simulink model "Trajectories_Transpalet"  (R2022a)
settings: Solver=VariableStepAuto  StartTime=0.0  StopTime=10.0  RelTol=1e-3
libraries: roblocks x1, simulink x1
settings Model: Creator=antonio  LastModifiedBy=antonio

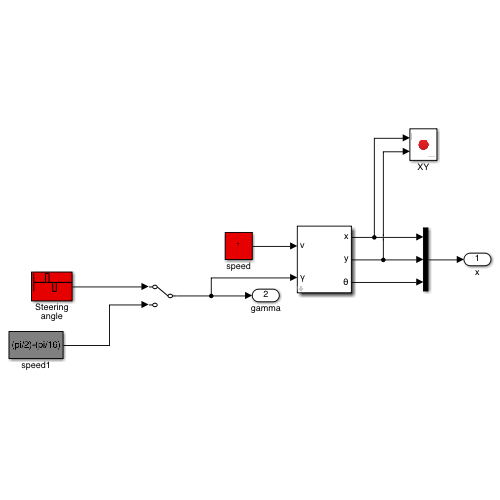
[thumbnail: Simulink's stored preview of the top-level diagram]
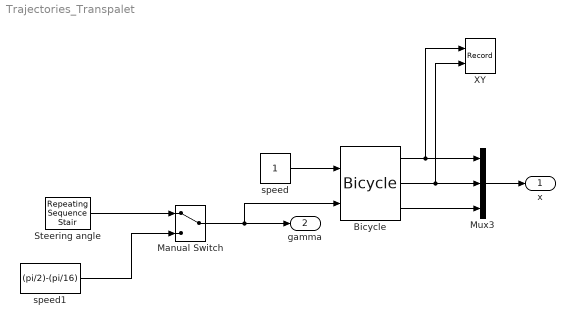
== system Trajectories_Transpalet ==
  Bicycle : roblocks/Vehicles/Bicycle  vlim=1  accel=Inf  alim=pi/2  steer_rate=Inf  L=1  x0=[0, 0, 0]
  Manual Switch : ManualSwitch
  Mux3 : Mux  Inputs=3
  Steering angle : simulink/Sources/Repeating Sequence Stair  OutValues=[0 0 0 0.5 0 -0.5 0 0 0 0]  tsamp=1  OutMin=[]  OutMax=[]  OutDataTypeStr=double  OutputDataTypeScalingMode=Specify via dialog  OutDataType=double  ConRadixGroup=Best Precision: Vector-wise  OutScaling=2^-12
  XY : Record  VariableName=recorout  RecordToWorkspace=on  FileSettingsInternal="{\"entries\":[{\"content\":{\"excelSettings\":{\"content\":{},\"type\":\"Streamout.ExcelSettings\"}},\"type\":\"Streamout.FileSettingStorage\",\"uuid\":\"5e76ab6b-3c48-49bd-98b9-b0ca941eaadb\"}],\"packageUris\":[\"http://schema.mathworks.com/mf0/streamout_blocks/R2020a\"],\"version\":\"1.0\"}"  Layout=[1 1]  SignalsInternal="{\"entries\":[{\"content\":{\"signals\":[{\"content\":{\"blockPath\":[\"Trajectories_Transpalet/XY\"],\"channel\":[],\"dimensions\":[1],\"domain\":\"Trajectories_Transpalet/XY\",\"lineColor\":\"#ff6929\",\"plots\":[1],\"port\":1,\"sid\":[\"\"],\"signalID\":1505,\"signalName\":\"Bicycle:1\"},\"type\":\"RecordBlkView.Signal\",\"uuid\":\"bba8ad1c-b6cc-4c10-82e1-d9e8909c4ac5\"},{\"content\":{\"blockPath\":[\"Trajectories_Transpalet/XY\"],\"channel\":[],\"dimensions\":[1],\"domain\":\"Trajectories_Transpalet/XY\",\"lineColor\":\"#b746ff\",\"plots\":[1],\"port\":2,\"sid\":[\"\"],\"signalID\":1509,\"signalName\":\"Bicycle:2\"},\"type\":\"RecordBlkView.Signal\",\"uuid\":\"132b81f0-6149-414a-8851-04aafb605e0d\"}]},\"type\":\"RecordBlkView.InputSignals\",\"uuid\":\"d89f0194-8b88-4c9a-aee1-29982656cbe6\"}],\"packageUris\":[\"http://schema.mathworks.com/mf0/streamout_blocks/R2020a\"],\"version\":\"1.0\"}"  VisualizationBindings="{\"xyplotplugin\":{\"info\":[{\"series\":[],\"subplotID\":1}]}}"  CompatibilityTag=XY  st=-1
  speed : Constant  VectorParams1D=off  SampleTime=0.02
  speed1 : Constant  Value=(pi/2)-(pi/16)  VectorParams1D=off  SampleTime=0.02
  x : Outport
  gamma : Outport  Port=2
  wires:
  Mux3/1 -> x/1
  Bicycle/2 -> Mux3/2, XY/2
  Bicycle/1 -> XY/1, Mux3/1
  Bicycle/3 -> Mux3/3
  speed/1 -> Bicycle/1
  Steering angle/1 -> Manual Switch/1
  Manual Switch/1 -> Bicycle/2, gamma/1
  speed1/1 -> Manual Switch/2
